simulink model "assign"  (Simulink 8.4)
settings: Solver=ode45  StartTime=0.0  StopTime=110  RelTol=1e-3
libraries: simulink x2
CloseFcn:
  | rtwprivate ssgensfun ModelCloseRequest nlgentpl
settings Model: Creator=lbusoniu  LastModifiedBy=Steven  ExtModeAutoUpdateStatusClock=off  BufferReuse=off
settings DataIOCC: SaveOutput=off  SaveTime=off  SignalLoggingName=sigsOut
settings OptimizationCC: OptimizeBlockIOStorage=off  BufferReuse=off  GlobalBufferReuse=off  ExpressionFolding=off  ExpressionDepthLimit=128  LocalBlockOutputs=off  InitFltsAndDblsToZero=on
settings DebuggingCC: SaveWithParameterizedLinksMsg=none  SignalResolutionControl=TryResolveAllWithWarning  SolverPrmCheckMsg=none  MultiTaskDSMMsg=warning  MultiTaskCondExecSysMsg=none  StateNameClashWarn=none
settings HardwareCC: TargetUnknown=on
settings RTWCC: IncludeERTFirstTime=on
settings GRTTargetCC: TargetFcnLib=ansi_tfl_tmw.mat

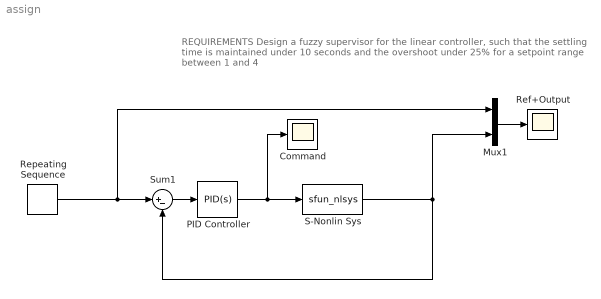
== system assign ==
  note: REQUIREMENTS
      | Design a fuzzy supervisor for the linear controller, such that
      | the settling time is maintained under 10 seconds and the overshoot under 25%
      | for a setpoint range between 1 and 4
  Command : Scope
      settings: TimeRange=120  YMin=-0.05  YMax=0.15  SaveName=u
  Mux1 : Mux  Inputs=2
  PID Controller : simulink/Continuous/PID Controller  Controller=PID  TimeDomain=Continuous-time  SampleTime=-1  IntegratorMethod=Forward Euler  FilterMethod=Forward Euler  Form=Parallel  P=0.04  I=0  D=0.1  N=100  InitialConditionSource=internal  InitialConditionForIntegrator=0  InitialConditionForFilter=0  ExternalReset=none  LimitOutput=off  UpperSaturationLimit=inf  LowerSaturationLimit=-inf  LinearizeAsGain=on  AntiWindupMode=none  Kb=1  TrackingMode=off  Kt=1  PParamMin=[]  PParamMax=[]  IParamMin=[]  IParamMax=[]  DParamMin=[]  DParamMax=[]  NParamMin=[]  NParamMax=[]  KbParamMin=[]  KbParamMax=[]  KtParamMin=[]  KtParamMax=[]  POutMin=[]  POutMax=[]  IOutMin=[]  IOutMax=[]  DOutMin=[]  DOutMax=[]  NOutMin=[]  NOutMax=[]  KbOutMin=[]  KbOutMax=[]  KtOutMin=[]  KtOutMax=[]  IntegratorOutMin=[]  IntegratorOutMax=[]  FilterOutMin=[]  FilterOutMax=[]  SumOutMin=[]  SumOutMax=[]  SumI1OutMin=[]  SumI1OutMax=[]  SumI2OutMin=[]  SumI2OutMax=[]  SumI3OutMin=[]  SumI3OutMax=[]  SumDOutMin=[]  SumDOutMax=[]  SaturationOutMin=[]  SaturationOutMax=[]  IntegratorContinuousStateAttributes=''  IntegratorStateMustResolveToSignalObject=off  IntegratorRTWStateStorageClass=Auto  FilterContinuousStateAttributes=''  FilterStateMustResolveToSignalObject=off  FilterRTWStateStorageClass=Auto  DifferentiatorICPrevScaledInput=0  DifferentiatorOutMin=[]  DifferentiatorOutMax=[]  UseFilter=on
  Ref+Output : Scope
      settings: TimeRange=120  YMin=0  SaveName=u2
  Repeating Sequence : simulink/Sources/Repeating Sequence  rep_seq_t=[0 15 15.5 30 30.5 45 45.5 60 60.5 75 75.5 90 91.5 111]  rep_seq_y=[1 1 .5 .5 2 2 1.5 1.5 3 3 2.5 2.5 4 4]
  S-Nonlin Sys : S-Function  FunctionName=sfun_nlsys  EnableBusSupport=off
  Sum1 : Sum  Inputs=|+-  SaturateOnIntegerOverflow=on
  wires:
  Sum1/1 -> PID Controller/1
  S-Nonlin Sys/1 -> Sum1/2, Mux1/2
  PID Controller/1 -> S-Nonlin Sys/1, Command/1
  Mux1/1 -> Ref+Output/1
  Repeating Sequence/1 -> Sum1/1, Mux1/1
